simulink model "segundoboceto"  (R2017a)
settings: Solver=ode3  StartTime=0.0  StopTime=6.3  FixedStep=5e-3  RelTol=1e-3
values from neighbouring files (symbols this model uses):
  L1 = L1/100    [calculodepar.m]
  L2 = L2/100    [calculodepar.m]
  m = 6    [calculodepar.m]
  N = m*g - ten*sin(beta)    [calculodepar.m]    (also in main.m = 360)
undefined symbols (not defined in the file or in its folder): correderaconcaja, pasador0, RootGround, RootPart, segundoboceto
libraries: mblibv1 x15
settings Model: Creator=angel  LastModifiedBy=angel
settings SimMechanicsCC: VisOnUpdateDiagram=on  VisDuringSimulation=on

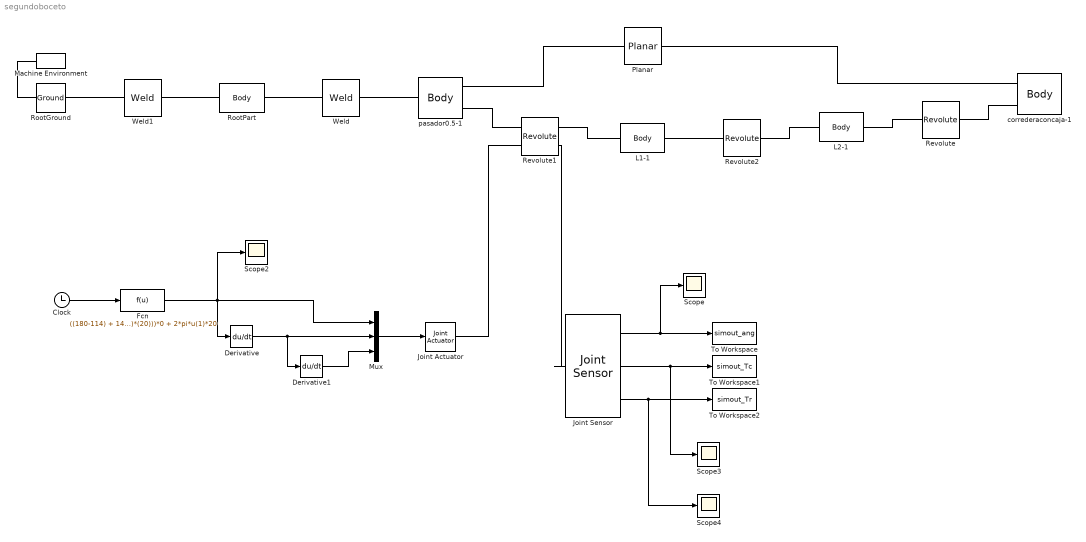
== system segundoboceto ==
  Clock : Clock
  Derivative : Derivative
  Derivative1 : Derivative
  Fcn : Fcn  Expr=((180-114) + 14*sin(2*pi*u(1)*(20)))*0 + 2*pi*u(1)*20
  Joint Actuator : mblibv1/Sensors &  Actuators/Joint Actuator  UpdateFromCAD=off  PhysicalDomain=Mechanical  PortType=blob  ActuationStyle=Motion  AngleUnits=deg  ArcVelocityUnits=deg/s  ArcAccelerationUnits=deg/s^2  CoordPositionUnits=m  VelocityUnits=m/s  AccelerationUnits=m/s^2  ForceUnits=N  TorqueUnits=N*m  ActiveIO=on  Width=3  DialogClass=MechanicalActuatorBlock  Primitive=R1  ReferenceFrame=Absolute (World)
      settings: SourceProductName=Simscape Multibody  SourceProductBaseCode=MS
  Joint Sensor : mblibv1/Sensors &  Actuators/Joint Sensor  UpdateFromCAD=off  PhysicalDomain=Mechanical  PortType=blob  Muxed=off  Pose=off  Angle=on  AngleUnits=deg  ArcVelocity=off  ArcVelocityUnits=deg/s  ArcAcceleration=off  ArcAccelerationUnits=deg/s^2  CoordPosition=on  CoordPositionUnits=m  Velocity=off  VelocityUnits=m/s  Acceleration=off  AccelerationUnits=m/s^2  Quaternion=on  QuaternionDT=off  QuaternionDDT=off  QuaternionUnits=off  OutputVector=[1]  ActiveIO=on  Width=5  DialogClass=MechanicalSensorBlock  Primitive=R1  Force=off  ForceUnits=N  Torque=on  TorqueUnits=N*m  ReferenceFrame=Absolute (World)  ReactionSensedSide=Base  ReactionReferenceFrame=Absolute (World)  ReactionForce=off  ReactionForceUnits=N  ReactionMoment=on  ReactionMomentUnits=N*m
      settings: SourceProductName=Simscape Multibody  SourceProductBaseCode=MS
  L1-1 : mblibv1/Bodies/Body  LConnTagsString=CS2  RConnTagsString=CS3  UpdateFromCAD=on  PMImportedID=L1-1  DialogClass=MechanicalBodyBlock  Mass=0.00593014  MassUnits=kg  InertiaUnits=kg*m^2  Inertia=[1.04021e-06,0,0;0,1.07865e-06,0;0,0,6.31529e-08]  Shape=Cylinder  ShapeDims=[1 1]  ShapeUnits=m  ShapeUse=false  Density=1  DensityUnits=kg/m^3  DensityUse=false  GraphicsMode=GFXFILE  GraphicsFileName=segundoboceto - L1-1.STL  BodyColorSelMode=COLORPALETTE  BodyColor=[0.666667;0.698039;0.768627]  AttachedToCS=CS1  CG=Right$CG$[-0.0264101 -0.000554302 0.00308157]$WORLD$WORLD$m$[0.345922 0 0.938263;0 1 0;-0.938263 0 0.345922]$3x3 Transform$rad$WORLD$false$L1-1::CG(AUTOGEN)  WorkingFrames=Right$CS1$[-0.0076448 -0.0030543 0.01]$WORLD$WORLD$m$[0.345922 0 0.938263;0 1 0;-0.938263 0 0.345922]$3x3 Transform$rad$WORLD$false$L1-1::CS1(AUTOGEN)#Left$CS2$[-0.0076448 -0.0030543 0.01]$WORLD$WORLD$m$[1 0 0;0 1 0;0 0 1]$3x3 Transform$rad$WORLD$true$L1-1:-:pasador0.5-1::L1-1(AUTOGEN)#Right$CS3$[-0.0451753 0.0019457 -0.00383687]$WORLD$WORLD$m$[1 0 0;0 1 0;0 0 1]$3x3 Transform$rad$WORLD$true$L1-1:-:L2-1::L1-1(AUTOGEN)  CGPos=[-0.0264101 -0.000554302 0.00308157]  CGRot=[0.345922 0 0.938263;0 1 0;-0.938263 0 0.345922]  CS0Pos=[]  CS0Rot=[]  CS1Pos=[-0.0076448 -0.0030543 0.01]  CS1Rot=[0.345922 0 0.938263;0 1 0;-0.938263 0 0.345922]  CS2Pos=[-0.0076448 -0.0030543 0.01]  CS2Rot=[1 0 0;0 1 0;0 0 1]  CS3Pos=[-0.0451753 0.0019457 -0.00383687]  CS3Rot=[1 0 0;0 1 0;0 0 1]  CS4Pos=[]  CS4Rot=[]  CS5Pos=[]  CS5Rot=[]  CS6Pos=[]  CS6Rot=[]  CS7Pos=[]  CS7Rot=[]  CS8Pos=[]  CS8Rot=[]  CS9Pos=[]  CS9Rot=[]  CS10Pos=[]  CS10Rot=[]  CS11Pos=[]  CS11Rot=[]  CS12Pos=[]  CS12Rot=[]  CS13Pos=[]  CS13Rot=[]  CS14Pos=[]  CS14Rot=[]  CS15Pos=[]  CS15Rot=[]  CS16Pos=[]  CS16Rot=[]  CS17Pos=[]  CS17Rot=[]  CS18Pos=[]  CS18Rot=[]  CS19Pos=[]  CS19Rot=[]  CS20Pos=[]  CS20Rot=[]
      settings: SourceProductName=Simscape Multibody  SourceProductBaseCode=MS
  L2-1 : mblibv1/Bodies/Body  LConnTagsString=CS3  RConnTagsString=CS2  UpdateFromCAD=on  PMImportedID=L2-1  DialogClass=MechanicalBodyBlock  Mass=0.00998014  MassUnits=kg  InertiaUnits=kg*m^2  Inertia=[4.69227e-06,0,0;0,4.75602e-06,0;0,0,1.0534e-07]  Shape=Cylinder  ShapeDims=[1 1]  ShapeUnits=m  ShapeUse=false  Density=1  DensityUnits=kg/m^3  DensityUse=false  GraphicsMode=GFXFILE  GraphicsFileName=segundoboceto - L2-1.STL  BodyColorSelMode=COLORPALETTE  BodyColor=[0.898039;0.917647;0.929412]  AttachedToCS=CS1  CG=Right$CG$[-0.0264101 0.0044457 -0.0333812]$WORLD$WORLD$m$[0.844122 0 -0.53615;0 1 0;0.53615 0 0.844122]$3x3 Transform$rad$WORLD$false$L2-1::CG(AUTOGEN)  WorkingFrames=Right$CS1$[-0.0451753 0.0019457 -0.00383687]$WORLD$WORLD$m$[0.844122 0 -0.53615;0 1 0;0.53615 0 0.844122]$3x3 Transform$rad$WORLD$false$L2-1::CS1(AUTOGEN)#Right$CS2$[-0.0076448 0.0069457 -0.0629254]$WORLD$WORLD$m$[1 0 0;0 1 0;0 0 1]$3x3 Transform$rad$WORLD$true$L2-1:-:correderaconcaja-1::L2-1(AUTOGEN)#Left$CS3$[-0.0451753 0.0019457 -0.00383687]$WORLD$WORLD$m$[1 0 0;0 1 0;0 0 1]$3x3 Transform$rad$WORLD$true$L1-1:-:L2-1::L2-1(AUTOGEN)  CGPos=[-0.0264101 0.0044457 -0.0333812]  CGRot=[0.844122 0 -0.53615;0 1 0;0.53615 0 0.844122]  CS0Pos=[]  CS0Rot=[]  CS1Pos=[-0.0451753 0.0019457 -0.00383687]  CS1Rot=[0.844122 0 -0.53615;0 1 0;0.53615 0 0.844122]  CS2Pos=[-0.0076448 0.0069457 -0.0629254]  CS2Rot=[1 0 0;0 1 0;0 0 1]  CS3Pos=[-0.0451753 0.0019457 -0.00383687]  CS3Rot=[1 0 0;0 1 0;0 0 1]  CS4Pos=[]  CS4Rot=[]  CS5Pos=[]  CS5Rot=[]  CS6Pos=[]  CS6Rot=[]  CS7Pos=[]  CS7Rot=[]  CS8Pos=[]  CS8Rot=[]  CS9Pos=[]  CS9Rot=[]  CS10Pos=[]  CS10Rot=[]  CS11Pos=[]  CS11Rot=[]  CS12Pos=[]  CS12Rot=[]  CS13Pos=[]  CS13Rot=[]  CS14Pos=[]  CS14Rot=[]  CS15Pos=[]  CS15Rot=[]  CS16Pos=[]  CS16Rot=[]  CS17Pos=[]  CS17Rot=[]  CS18Pos=[]  CS18Rot=[]  CS19Pos=[]  CS19Rot=[]  CS20Pos=[]  CS20Rot=[]
      settings: SourceProductName=Simscape Multibody  SourceProductBaseCode=MS
  Machine Environment : mblibv1/Bodies/Machine Environment  PortType=env  PhysicalDomain=Mechanical  DialogTemplateClass=MECH.MachineEnvironment  SyncWhenCopied=off  Gravity=[0 -9.81 0]  GravityUnits=m/s^2  GravityAsSignal=off  Dimensionality=Auto-detect  AnalysisType=Forward dynamics  LinearAssemblyTolerance=1e-3  LinearAssemblyToleranceUnits=m  AngularAssemblyTolerance=1e-3  AngularAssemblyToleranceUnits=rad  ConstraintSolverType=Stabilizing  ConstraintRelTolerance=1e-4  ConstraintAbsTolerance=1e-4  UseRobustSingularityHandling=off  RedundancyAnalysisToleranceType=Automatically select tolerance  RedundancyAnalysisTolerance=1e-14  StatePerturbationType=Fixed  PerturbationSize=1e-5  VisualizeMachine=on  BodyVisualizationType=Use model default body geometries  BodyColorSelMode=Use model default  DefaultBodyColor=[1 0 0]
      settings: SourceProductName=Simscape Multibody  SourceProductBaseCode=MS
  Mux : Mux  Inputs=3
  Planar : mblibv1/Joints/Planar  LConnTagsString=__newl0  RConnTagsString=__newr0  UpdateFromCAD=on  PMImportedID=correderaconcaja-1:-:pasador0.5-1  NumSAPorts=0  CutJoint=off  MarkAsCut=off  Primitives=prismatic_prismatic  PrimitiveProps=P1$WORLD$[0,1,0]$prismatic#P2$WORLD$[0,0,1]$prismatic#R1$WORLD$[-1,0,0]$revolute  DialogClass=JointBlock  P1Axis=[0,1,0]  P2Axis=[0,0,1]  R1Axis=[-1,0,0]
      settings: SourceProductName=Simscape Multibody  SourceProductBaseCode=MS
  Revolute : mblibv1/Joints/Revolute  LConnTagsString=__newl0  RConnTagsString=__newr0  UpdateFromCAD=on  PMImportedID=L2-1:-:correderaconcaja-1  NumSAPorts=0  CutJoint=off  MarkAsCut=off  Primitives=prismatic  PrimitiveProps=R1$WORLD$[0,1,0]$revolute  DialogClass=JointBlock  R1Axis=[0,1,0]
      settings: SourceProductName=Simscape Multibody  SourceProductBaseCode=MS
  Revolute1 : mblibv1/Joints/Revolute  LConnTagsString=__newl0|SA1  RConnTagsString=__newr0|SA1  UpdateFromCAD=on  PMImportedID=L1-1:-:pasador0.5-1  NumSAPorts=2  CutJoint=off  MarkAsCut=off  Primitives=prismatic  PrimitiveProps=R1$World$[0,-1,0]$revolute  DialogClass=JointBlock  R1Axis=[0,-1,0]
      settings: SourceProductName=Simscape Multibody  SourceProductBaseCode=MS
  Revolute2 : mblibv1/Joints/Revolute  LConnTagsString=__newl0  RConnTagsString=__newr0  UpdateFromCAD=on  PMImportedID=L1-1:-:L2-1  NumSAPorts=0  CutJoint=off  MarkAsCut=off  Primitives=prismatic  PrimitiveProps=R1$WORLD$[0,1,0]$revolute  DialogClass=JointBlock  R1Axis=[0,1,0]
      settings: SourceProductName=Simscape Multibody  SourceProductBaseCode=MS
  RootGround : mblibv1/Bodies/Ground  UpdateFromCAD=on  PMImportedID=RootGround  LeftPortType=env  RightPortType=workingframe  PhysicalDomain=Mechanical  DialogClass=GroundBlock  CoordPosition=[-0.00770419,-0.015352,-0.220462]  CoordPositionUnits=m  StateVectorMgrId=0  MachineId=[1 0]  ShowEnvPort=on  ParameterChecksum=[3562357946, 157376236, 2861734617, 1544863643]  TopologyChecksum=[639002679, 929810166, 2874059122, 217083452]
      settings: SourceProductName=Simscape Multibody  SourceProductBaseCode=MS
  RootPart : mblibv1/Bodies/Body  LConnTagsString=CS3  RConnTagsString=CS2  UpdateFromCAD=on  PMImportedID=segundoboceto/RootPart  DialogClass=MechanicalBodyBlock  Mass=0  MassUnits=kg  InertiaUnits=kg*m^2  Inertia=[0,0,0;0,0,0;0,0,0]  Shape=Cylinder  ShapeDims=[1 1]  ShapeUnits=m  ShapeUse=false  Density=1  DensityUnits=kg/m^3  DensityUse=false  GraphicsMode=MACHINE_DEFAULT  BodyColorSelMode=MACHINE_DEFAULT  BodyColor=[1;0;0]  AttachedToCS=CS1  CG=Right$CG$[-0.00770419 -0.015352 -0.220462]$WORLD$WORLD$m$[1 0 0;0 1 0;0 0 1]$3x3 Transform$rad$WORLD$false$segundoboceto/RootPart::CG(AUTOGEN)  WorkingFrames=Right$CS1$[0 0 0]$WORLD$WORLD$m$[1 0 0;0 1 0;0 0 1]$3x3 Transform$rad$WORLD$false$segundoboceto/RootPart::CS1(AUTOGEN)#Right$CS2$[0.00420889 0.0019457 -0.0842636]$WORLD$WORLD$m$[1 0 0;0 1 0;0 0 1]$3x3 Transform$rad$WORLD$true$pasador0.5-1:-:segundoboceto/RootPart::segundoboceto/RootPart(AUTOGEN)#Left$CS3$[-0.00770419 -0.015352 -0.220462]$WORLD$WORLD$m$[1 0 0;0 1 0;0 0 1]$3x3 Transform$rad$WORLD$true$RootGround:-:segundoboceto/RootPart::segundoboceto/RootPart(AUTOGEN)  CGPos=[-0.00770419 -0.015352 -0.220462]  CGRot=[1 0 0;0 1 0;0 0 1]  CS0Pos=[]  CS0Rot=[]  CS1Pos=[0 0 0]  CS1Rot=[1 0 0;0 1 0;0 0 1]  CS2Pos=[0.00420889 0.0019457 -0.0842636]  CS2Rot=[1 0 0;0 1 0;0 0 1]  CS3Pos=[-0.00770419 -0.015352 -0.220462]  CS3Rot=[1 0 0;0 1 0;0 0 1]  CS4Pos=[]  CS4Rot=[]  CS5Pos=[]  CS5Rot=[]  CS6Pos=[]  CS6Rot=[]  CS7Pos=[]  CS7Rot=[]  CS8Pos=[]  CS8Rot=[]  CS9Pos=[]  CS9Rot=[]  CS10Pos=[]  CS10Rot=[]  CS11Pos=[]  CS11Rot=[]  CS12Pos=[]  CS12Rot=[]  CS13Pos=[]  CS13Rot=[]  CS14Pos=[]  CS14Rot=[]  CS15Pos=[]  CS15Rot=[]  CS16Pos=[]  CS16Rot=[]  CS17Pos=[]  CS17Rot=[]  CS18Pos=[]  CS18Rot=[]  CS19Pos=[]  CS19Rot=[]  CS20Pos=[]  CS20Rot=[]
      settings: SourceProductName=Simscape Multibody  SourceProductBaseCode=MS
  Scope{,2..4} (4 alike) : Scope
  To Workspace : ToWorkspace  VariableName=simout_ang  SaveFormat=Timeseries  SampleTime=-1
  To Workspace1 : ToWorkspace  VariableName=simout_Tc  SaveFormat=Timeseries  SampleTime=-1
  To Workspace2 : ToWorkspace  VariableName=simout_Tr  SaveFormat=Timeseries  SampleTime=-1
  Weld : mblibv1/Joints/Weld  LConnTagsString=__newl0  RConnTagsString=__newr0  UpdateFromCAD=on  PMImportedID=pasador0.5-1:-:segundoboceto/RootPart  NumSAPorts=0  CutJoint=off  MarkAsCut=off  Primitives=weld  PrimitiveProps=W$WORLD$[0.57735,0.57735,0.57735]$weld  DialogClass=JointBlock  WAxis=[0.57735,0.57735,0.57735]
      settings: SourceProductName=Simscape Multibody  SourceProductBaseCode=MS
  Weld1 : mblibv1/Joints/Weld  LConnTagsString=__newl0  RConnTagsString=__newr0  UpdateFromCAD=on  PMImportedID=RootGround:-:segundoboceto/RootPart  NumSAPorts=0  CutJoint=off  MarkAsCut=off  Primitives=weld  PrimitiveProps=W$WORLD$[0.57735,0.57735,0.57735]$weld  DialogClass=JointBlock  WAxis=[0.57735,0.57735,0.57735]
      settings: SourceProductName=Simscape Multibody  SourceProductBaseCode=MS
  correderaconcaja-1 : mblibv1/Bodies/Body  LConnTagsString=CS2|CS3  UpdateFromCAD=on  PMImportedID=correderaconcaja-1  DialogClass=MechanicalBodyBlock  Mass=2.20599  MassUnits=kg  InertiaUnits=kg*m^2  Inertia=[0.0276771,0,0;0,0.0505932,2.00009e-05;0,2.00009e-05,0.0275225]  Shape=Cylinder  ShapeDims=[1 1]  ShapeUnits=m  ShapeUse=false  Density=1  DensityUnits=kg/m^3  DensityUse=false  GraphicsMode=GFXFILE  GraphicsFileName=segundoboceto - correderaconcaja-1.STL  BodyColorSelMode=COLORPALETTE  BodyColor=[0.898039;0.917647;0.929412]  AttachedToCS=CS1  CG=Right$CG$[-0.0076448 -0.015591 -0.222773]$WORLD$WORLD$m$[-1 0 0;0 1 0;0 0 -1]$3x3 Transform$rad$WORLD$false$correderaconcaja-1::CG(AUTOGEN)  WorkingFrames=Right$CS1$[-0.0076448 0.0044457 -0.0729254]$WORLD$WORLD$m$[-1 0 0;0 1 0;0 0 -1]$3x3 Transform$rad$WORLD$false$correderaconcaja-1::CS1(AUTOGEN)#Left$CS2$[-0.0026448 0.0069457 -0.104995]$WORLD$WORLD$m$[1 0 0;0 1 0;0 0 1]$3x3 Transform$rad$WORLD$true$correderaconcaja-1:-:pasador0.5-1::correderaconcaja-1(AUTOGEN)#Left$CS3$[-0.0076448 0.0069457 -0.0629254]$WORLD$WORLD$m$[1 0 0;0 1 0;0 0 1]$3x3 Transform$rad$WORLD$true$L2-1:-:correderaconcaja-1::correderaconcaja-1(AUTOGEN)  CGPos=[-0.0076448 -0.015591 -0.222773]  CGRot=[-1 0 0;0 1 0;0 0 -1]  CS0Pos=[]  CS0Rot=[]  CS1Pos=[-0.0076448 0.0044457 -0.0729254]  CS1Rot=[-1 0 0;0 1 0;0 0 -1]  CS2Pos=[-0.0026448 0.0069457 -0.104995]  CS2Rot=[1 0 0;0 1 0;0 0 1]  CS3Pos=[-0.0076448 0.0069457 -0.0629254]  CS3Rot=[1 0 0;0 1 0;0 0 1]  CS4Pos=[]  CS4Rot=[]  CS5Pos=[]  CS5Rot=[]  CS6Pos=[]  CS6Rot=[]  CS7Pos=[]  CS7Rot=[]  CS8Pos=[]  CS8Rot=[]  CS9Pos=[]  CS9Rot=[]  CS10Pos=[]  CS10Rot=[]  CS11Pos=[]  CS11Rot=[]  CS12Pos=[]  CS12Rot=[]  CS13Pos=[]  CS13Rot=[]  CS14Pos=[]  CS14Rot=[]  CS15Pos=[]  CS15Rot=[]  CS16Pos=[]  CS16Rot=[]  CS17Pos=[]  CS17Rot=[]  CS18Pos=[]  CS18Rot=[]  CS19Pos=[]  CS19Rot=[]  CS20Pos=[]  CS20Rot=[]
      settings: SourceProductName=Simscape Multibody  SourceProductBaseCode=MS
  pasador0.5-1 : mblibv1/Bodies/Body  LConnTagsString=CS2  RConnTagsString=CS3|CS4  UpdateFromCAD=on  PMImportedID=pasador0.5-1  DialogClass=MechanicalBodyBlock  Mass=0.0139846  MassUnits=kg  InertiaUnits=kg*m^2  Inertia=[6.31237e-06,0,6.15708e-07;0,6.51445e-06,0;6.15708e-07,0,4.3515e-07]  Shape=Cylinder  ShapeDims=[1 1]  ShapeUnits=m  ShapeUse=false  Density=1  DensityUnits=kg/m^3  DensityUse=false  GraphicsMode=GFXFILE  GraphicsFileName=segundoboceto - pasador0.5-1.STL  BodyColorSelMode=COLORPALETTE  BodyColor=[0.898039;0.917647;0.929412]  AttachedToCS=CS1  CG=Right$CG$[0.00420889 0.0019457 -0.0842636]$WORLD$WORLD$m$[1 0 0;0 1 0;0 0 1]$3x3 Transform$rad$WORLD$false$pasador0.5-1::CG(AUTOGEN)  WorkingFrames=Right$CS1$[-0.0076448 -0.0030543 0.01]$WORLD$WORLD$m$[1 0 0;0 1 0;0 0 1]$3x3 Transform$rad$WORLD$false$pasador0.5-1::CS1(AUTOGEN)#Left$CS2$[0.00420889 0.0019457 -0.0842636]$WORLD$WORLD$m$[1 0 0;0 1 0;0 0 1]$3x3 Transform$rad$WORLD$true$pasador0.5-1:-:segundoboceto/RootPart::pasador0.5-1(AUTOGEN)#Right$CS3$[-0.0026448 0.0069457 -0.104995]$WORLD$WORLD$m$[1 0 0;0 1 0;0 0 1]$3x3 Transform$rad$WORLD$true$correderaconcaja-1:-:pasador0.5-1::pasador0.5-1(AUTOGEN)#Right$CS4$[-0.0076448 -0.0030543 0.01]$WORLD$WORLD$m$[1 0 0;0 1 0;0 0 1]$3x3 Transform$rad$WORLD$true$L1-1:-:pasador0.5-1::pasador0.5-1(AUTOGEN)  CGPos=[0.00420889 0.0019457 -0.0842636]  CGRot=[1 0 0;0 1 0;0 0 1]  CS0Pos=[]  CS0Rot=[]  CS1Pos=[-0.0076448 -0.0030543 0.01]  CS1Rot=[1 0 0;0 1 0;0 0 1]  CS2Pos=[0.00420889 0.0019457 -0.0842636]  CS2Rot=[1 0 0;0 1 0;0 0 1]  CS3Pos=[-0.0026448 0.0069457 -0.104995]  CS3Rot=[1 0 0;0 1 0;0 0 1]  CS4Pos=[-0.0076448 -0.0030543 0.01]  CS4Rot=[1 0 0;0 1 0;0 0 1]  CS5Pos=[]  CS5Rot=[]  CS6Pos=[]  CS6Rot=[]  CS7Pos=[]  CS7Rot=[]  CS8Pos=[]  CS8Rot=[]  CS9Pos=[]  CS9Rot=[]  CS10Pos=[]  CS10Rot=[]  CS11Pos=[]  CS11Rot=[]  CS12Pos=[]  CS12Rot=[]  CS13Pos=[]  CS13Rot=[]  CS14Pos=[]  CS14Rot=[]  CS15Pos=[]  CS15Rot=[]  CS16Pos=[]  CS16Rot=[]  CS17Pos=[]  CS17Rot=[]  CS18Pos=[]  CS18Rot=[]  CS19Pos=[]  CS19Rot=[]  CS20Pos=[]  CS20Rot=[]
      settings: SourceProductName=Simscape Multibody  SourceProductBaseCode=MS
  wires:
  Derivative/1 -> Derivative1/1, Mux/2
  Joint Sensor/3 -> Scope4/1, To Workspace2/1
  Clock/1 -> Fcn/1
  Derivative1/1 -> Mux/3
  Mux/1 -> Joint Actuator/1
  Joint Sensor/1 -> Scope/1, To Workspace/1
  Fcn/1 -> Derivative/1, Mux/1, Scope2/1
  Joint Sensor/2 -> Scope3/1, To Workspace1/1
  connections:
  RootPart/RConn1 -- Weld/LConn1
  Weld/RConn1 -- pasador0.5-1/LConn1
  pasador0.5-1/RConn1 -- Planar/LConn1
  Planar/RConn1 -- correderaconcaja-1/LConn1
  L2-1/RConn1 -- Revolute/LConn1
  Revolute/RConn1 -- correderaconcaja-1/LConn2
  pasador0.5-1/RConn2 -- Revolute1/LConn1
  Revolute1/RConn1 -- L1-1/LConn1
  L1-1/RConn1 -- Revolute2/LConn1
  Revolute2/RConn1 -- L2-1/LConn1
  RootGround/RConn1 -- Weld1/LConn1
  Weld1/RConn1 -- RootPart/LConn1
  RootGround/LConn1 -- Machine Environment/RConn1
  Joint Sensor/LConn1 -- Revolute1/RConn2
  Joint Actuator/RConn1 -- Revolute1/LConn2
